simulink model "P3_model"  (R2023b)
settings: Solver=FixedStepAuto  StartTime=0.0  StopTime=240  FixedStep=0.01  RelTol=1e-3
values from neighbouring files (symbols this model uses):
  C0 = 0.0041    [init.m]
  C1 = 0.000066    (= 6.6e-05)    [init.m]
  C2 = 0.5*Rho*A*Cd    (= 0.51156)    [init.m]
  DriveData = DriveData_urban    [P3_runsim.m]
  Iw = 0.5*7*(r^2)    (= 0.4536)    [init.m]
  M = 1000    [init.m]
  mph2mps = 1600/3600    (= 0.444444444444)    [P3init.m]    (also in init.m)
  r = 0.36    [init.m]
  Time = (0:1:765)'    [init_HWY_DriveCycle.m]    (also in init_URB_DriveCycle.m = (0:1:1369)')
undefined symbols (not defined in the file or in its folder): carData
libraries: slpidlib x1
settings Model: Creator=anshu16  LastModifiedBy=jessi
settings SolverCC: AlgebraicLoopSolver=TrustRegion
settings OptimizationCC: ReuseModelBlockBuffer=off
settings DebuggingCC: UnconnectedInputMsg=warning  UnconnectedOutputMsg=warning  UnconnectedLineMsg=warning
settings ModelReferenceCC: EnableRefExpFcnMdlSchedulingChecks=on
settings SFSimCC: CustomCodeUndefinedFunction=UseInterfaceOnly

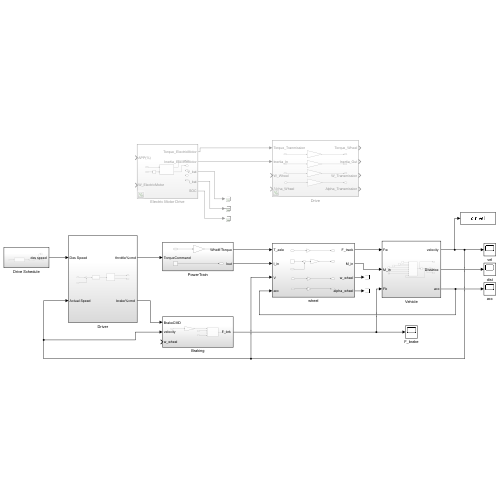
[thumbnail: Simulink's stored preview of the top-level diagram]
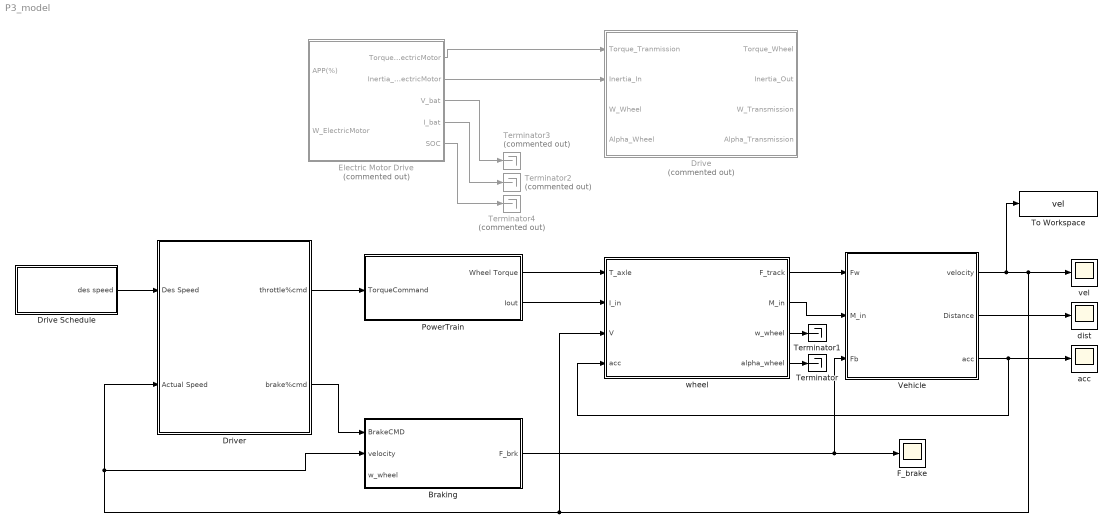
== system P3_model ==
  Braking : Subsystem
  Drive : Subsystem  Commented=on
  Drive Schedule : Subsystem
  "Driver " : Subsystem
  Electric Motor Drive : Subsystem  Commented=on
  F_brake : Scope
  PowerTrain : Subsystem
  Terminator : Terminator
  Terminator1 : Terminator
  Terminator2 : Terminator  Commented=on
  Terminator3 : Terminator  Commented=on
  Terminator4 : Terminator  Commented=on
  To Workspace : ToWorkspace  VariableName=vel  SaveFormat=Timeseries  SampleTime=-1
  Vehicle : Subsystem
  acc : Scope
  dist : Scope
  vel : Scope
  "wheel " : Subsystem
  wires:
  Drive Schedule/1("des speed ") -> "Driver "/1("Des Speed ")
  "Driver "/2("brake%cmd ") -> Braking/1("BrakeCMD ")
  Braking/1("F_brk ") -> Vehicle/3("Fb "), F_brake/1
  Vehicle/3(acc) -> acc/1, "wheel "/4(acc)
  PowerTrain/1(Wheel Torque) -> "wheel "/1(T_axle)
  PowerTrain/2(Iout) -> "wheel "/2(I_in)
  "wheel "/2(M_in) -> Vehicle/2("M_in ")
  "wheel "/1(F_track) -> Vehicle/1("Fw ")
  Vehicle/2("Distance ") -> dist/1
  Vehicle/1("velocity ") -> To Workspace/1, vel/1, "wheel "/3(V), "Driver "/2(Actual Speed), Braking/2("velocity ")
  "Driver "/1(throttle%cmd) -> PowerTrain/1(TorqueCommand)
  "wheel "/4(alpha_wheel) -> Terminator/1
  "wheel "/3(w_wheel) -> Terminator1/1
  Electric Motor Drive/3(V_bat) -> Terminator3/1
  Electric Motor Drive/4(I_bat) -> Terminator2/1
  Electric Motor Drive/5(SOC) -> Terminator4/1
  Electric Motor Drive/1(Torque_ElectricMotor) -> Drive/1(Torque_Tranmission)
  Electric Motor Drive/2(Inertia_ElectricMotor) -> Drive/2(Inertia_In)

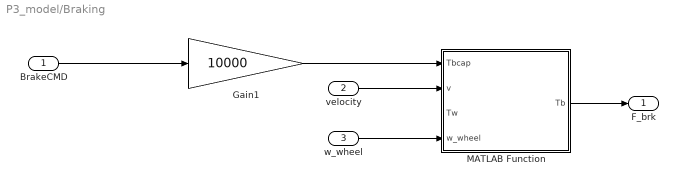
== system P3_model/Braking ==
  "BrakeCMD " : Inport
  "velocity " : Inport  Port=2
  w_wheel : Inport  Port=3
  Gain1 : Gain  Gain=10000
  MATLAB Function : MATLAB Function  TreatAsAtomicUnit=on
  "F_brk " : Outport  VectorParamsAs1DForOutWhenUnconnected=off
  wires:
  "BrakeCMD "/1 -> Gain1/1
  Gain1/1 -> MATLAB Function/1(Tbcap)
  MATLAB Function/1(Tb) -> "F_brk "/1
  "velocity "/1 -> MATLAB Function/2(v)
  w_wheel/1 -> MATLAB Function/4(w_wheel)

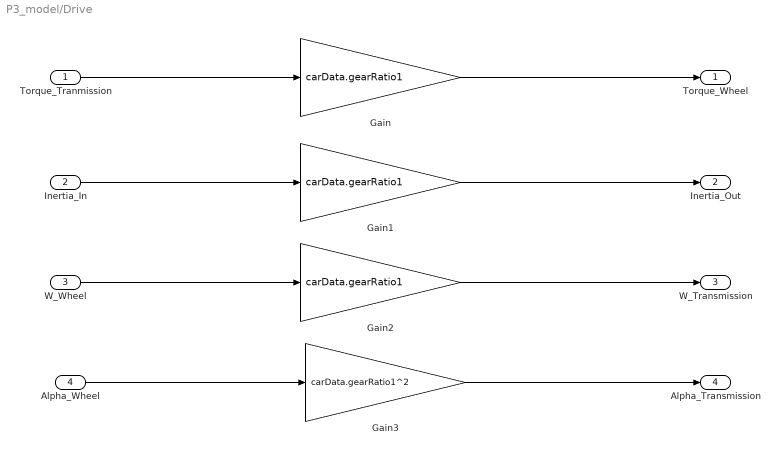
== system P3_model/Drive ==
  Torque_Tranmission : Inport
  Inertia_In : Inport  Port=2
  W_Wheel : Inport  Port=3
  Alpha_Wheel : Inport  Port=4
  Gain : Gain  Gain=carData.gearRatio1
  Gain1 : Gain  Gain=carData.gearRatio1
  Gain2 : Gain  Gain=carData.gearRatio1
  Gain3 : Gain  Gain=carData.gearRatio1^2
  Torque_Wheel : Outport
  Inertia_Out : Outport  Port=2
  W_Transmission : Outport  Port=3
  Alpha_Transmission : Outport  Port=4
  wires:
  Torque_Tranmission/1 -> Gain/1
  Inertia_In/1 -> Gain1/1
  W_Wheel/1 -> Gain2/1
  Alpha_Wheel/1 -> Gain3/1
  Gain/1 -> Torque_Wheel/1
  Gain1/1 -> Inertia_Out/1
  Gain2/1 -> W_Transmission/1
  Gain3/1 -> Alpha_Transmission/1

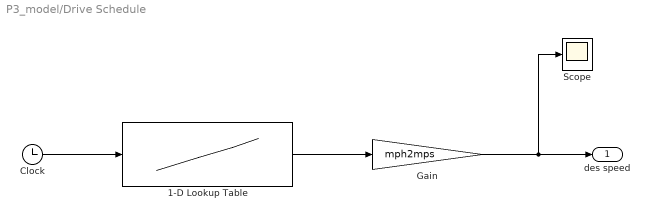
== system P3_model/Drive Schedule ==
  1-D Lookup Table : Lookup_n-D  NumberOfTableDimensions=1  BreakpointsForDimension1=Time  Table=DriveData  InternalRulePriority=Speed  RndMeth=Simplest
  Clock : Clock
  Gain : Gain  Gain=mph2mps
  Scope : Scope
  "des speed " : Outport  VectorParamsAs1DForOutWhenUnconnected=off
  wires:
  Clock/1 -> 1-D Lookup Table/1
  1-D Lookup Table/1 -> Gain/1
  Gain/1 -> "des speed "/1, Scope/1

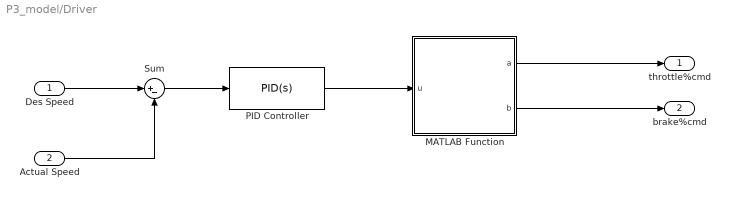
== system P3_model/Driver  ==
  "Des Speed " : Inport
  Actual Speed : Inport  Port=2
  MATLAB Function : MATLAB Function  TreatAsAtomicUnit=on
  PID Controller : slpidlib/PID Controller  Controller=PID  Form=Parallel  TimeDomain=Continuous-time  UseExternalTs=off  SampleTime=-1  IntegratorMethod=Forward Euler  FilterMethod=Forward Euler  ControllerParametersSource=internal  P=0.5  I=0  UseKiTs=off  D=0  N=100  UseFilter=on  TunerSelectOption=Transfer Function Based (PID Tuner App)  InitialConditionSource=internal  InitialConditionForIntegrator=0  InitialConditionForFilter=0  DifferentiatorICPrevScaledInput=0  ExternalReset=none  TrackingMode=off  Kt=1  LimitOutput=on  SatLimitsSource=internal  UpperSaturationLimit=1  LowerSaturationLimit=-1  LinearizeAsGain=off  AntiWindupMode=none  Kb=1  LimitIntegrator=off  UpperIntegratorSaturationLimit=inf  LowerIntegratorSaturationLimit=-inf  POutMin=[]  POutMax=[]  IOutMin=[]  IOutMax=[]  DOutMin=[]  DOutMax=[]  NOutMin=[]  NOutMax=[]  SumOutMin=[]  SumOutMax=[]  SaturationOutMin=[]  SaturationOutMax=[]  PParamMin=[]  PParamMax=[]  IParamMin=[]  IParamMax=[]  DParamMin=[]  DParamMax=[]  NParamMin=[]  NParamMax=[]  KbParamMin=[]  KbParamMax=[]  KtParamMin=[]  KtParamMax=[]  KbOutMin=[]  KbOutMax=[]  KtOutMin=[]  KtOutMax=[]  IntegratorOutMin=[]  IntegratorOutMax=[]  FilterOutMin=[]  FilterOutMax=[]  SumI1OutMin=[]  SumI1OutMax=[]  SumI2OutMin=[]  SumI2OutMax=[]  SumI3OutMin=[]  SumI3OutMax=[]  SumI4OutMin=[]  SumI4OutMax=[]  SumDOutMin=[]  SumDOutMax=[]  DifferentiatorOutMin=[]  DifferentiatorOutMax=[]  FilterDiffOutCoefMin=[]  FilterDiffOutCoefMax=[]  ReciprocalOutMin=[]  ReciprocalOutMax=[]  SumDenOutMin=[]  SumDenOutMax=[]  SumNumOutMin=[]  SumNumOutMax=[]  DivideOutMin=[]  DivideOutMax=[]  UdiffTsProdOutMin=[]  UdiffTsProdOutMax=[]  NTsProdOutMin=[]  NTsProdOutMax=[]  UintegralTsProdOutMin=[]  UintegralTsProdOutMax=[]  UngainTsProdOutMin=[]  UngainTsProdOutMax=[]  ClampingZeroOutDataTypeStr=Inherit: Inherit via back propagation  ClampingZeroOutMin=[]  ClampingZeroOutMax=[]  FilterDenConstantOutDataTypeStr=Inherit: Inherit via back propagation  FilterDenConstantOutMin=[]  FilterDenConstantOutMax=[]  PCopyOutDataTypeStr=Inherit: Inherit via back propagation  PCopyOutMin=[]  PCopyOutMax=[]  NCopyOutDataTypeStr=Inherit: Inherit via back propagation  NCopyOutMin=[]  NCopyOutMax=[]  IntegratorContinuousStateAttributes=''  IntegratorStateMustResolveToSignalObject=off  IntegratorRTWStateStorageClass=Auto  FilterContinuousStateAttributes=''  FilterStateMustResolveToSignalObject=off  FilterRTWStateStorageClass=Auto  ParallelPVariant=InternalParameters  IdealPVariant=Disabled  IVariant=InternalParameters  DVariant=InternalParameters  IntegratorVariant=Continuous  SatVariant=Enabled  AWVariant=Passthrough  PCopyVariant=Disabled  TRVariant=Disabled  FdbkBlocksVariant=Forward  IdealPFdbkVariant=Disabled  SatFdbkVariant=Disabled  DerivativeFilterVariant=ContFilter  NVariant=InternalParameters  NCopyVariant=Disabled  FilterICVariant=InternalICsFilter  IntegratorICVariant=InternalICs  ExternalResetVariant=Disabled  TRSumVariant=Passthrough  SumFdbkVariant=Disabled  SumVariant=Sum_PID  TsampFilterVariant=InternalTs  TsampNgainVariant=Passthrough  TsampIntegralVariant=Disabled_SignalSpec  ExternalSaturationOutDataTypeStr=Inherit: Same as second input
  Sum : Sum  Inputs=|+-
  throttle%cmd : Outport
  "brake%cmd " : Outport  Port=2
  wires:
  "Des Speed "/1 -> Sum/1
  Actual Speed/1 -> Sum/2
  MATLAB Function/2(b) -> "brake%cmd "/1
  MATLAB Function/1(a) -> throttle%cmd/1
  Sum/1 -> PID Controller/1
  PID Controller/1 -> MATLAB Function/1(u)

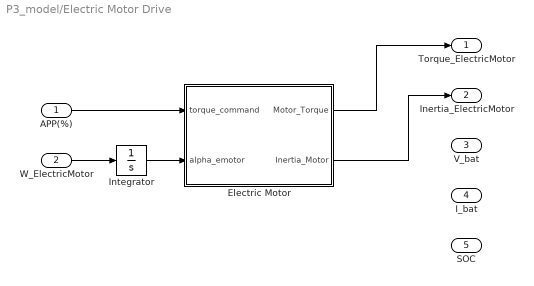
== system P3_model/Electric Motor Drive ==
  APP(%) : Inport
  W_ElectricMotor : Inport  Port=2
  Electric Motor : Subsystem
  Integrator : Integrator
  Torque_ElectricMotor : Outport
  Inertia_ElectricMotor : Outport  Port=2
  V_bat : Outport  Port=3
  I_bat : Outport  Port=4
  SOC : Outport  Port=5
  wires:
  Integrator/1 -> Electric Motor/2(alpha_emotor)
  W_ElectricMotor/1 -> Integrator/1
  APP(%)/1 -> Electric Motor/1(torque_command)
  Electric Motor/1(Motor_Torque) -> Torque_ElectricMotor/1
  Electric Motor/2(Inertia_Motor) -> Inertia_ElectricMotor/1

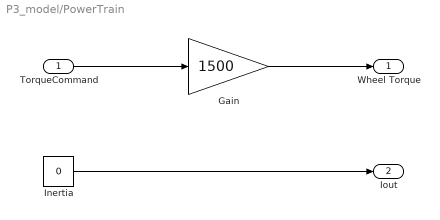
== system P3_model/PowerTrain ==
  TorqueCommand : Inport
  Gain : Gain  Gain=1500
  Inertia : Constant  Value=0
  Wheel Torque : Outport
  Iout : Outport  Port=2
  wires:
  TorqueCommand/1 -> Gain/1
  Gain/1 -> Wheel Torque/1
  Inertia/1 -> Iout/1

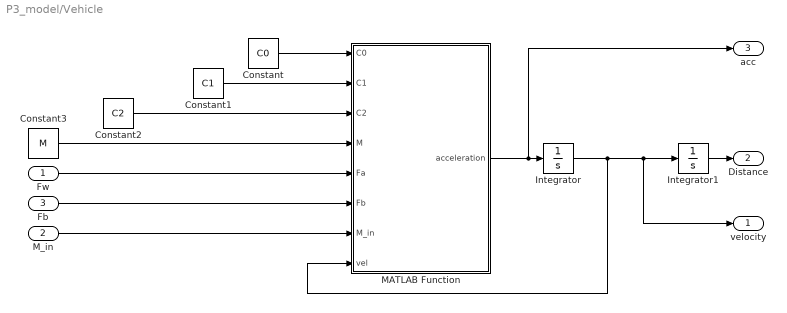
== system P3_model/Vehicle ==
  "Fw " : Inport
  "M_in " : Inport  Port=2
  "Fb " : Inport  Port=3
  Constant : Constant  Value=C0
  Constant1 : Constant  Value=C1
  Constant2 : Constant  Value=C2
  Constant3 : Constant  Value=M
  Integrator : Integrator  LimitOutput=on  LowerSaturationLimit=0
  Integrator1 : Integrator
  MATLAB Function : MATLAB Function  TreatAsAtomicUnit=on
  "velocity " : Outport  VectorParamsAs1DForOutWhenUnconnected=off
  "Distance " : Outport  Port=2  VectorParamsAs1DForOutWhenUnconnected=off
  acc : Outport  Port=3
  wires:
  Constant1/1 -> MATLAB Function/2(C1)
  Constant/1 -> MATLAB Function/1(C0)
  MATLAB Function/1(acceleration) -> acc/1, Integrator/1
  Constant2/1 -> MATLAB Function/3(C2)
  Constant3/1 -> MATLAB Function/4(M)
  "Fw "/1 -> MATLAB Function/5(Fa)
  "Fb "/1 -> MATLAB Function/6(Fb)
  Integrator/1 -> MATLAB Function/8(vel), "velocity "/1, Integrator1/1
  Integrator1/1 -> "Distance "/1
  "M_in "/1 -> MATLAB Function/7(M_in)

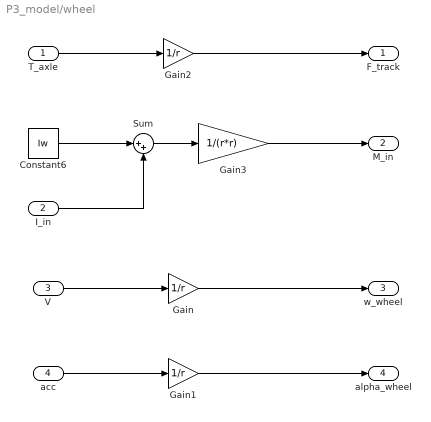
== system P3_model/wheel  ==
  T_axle : Inport
  I_in : Inport  Port=2
  V : Inport  Port=3
  acc : Inport  Port=4
  Constant6 : Constant  Value=Iw
  Gain : Gain  Gain=1/r
  Gain1 : Gain  Gain=1/r
  Gain2 : Gain  Gain=1/r
  Gain3 : Gain  Gain=1/(r*r)
  Sum : Sum  Inputs=|++
  F_track : Outport
  M_in : Outport  Port=2
  w_wheel : Outport  Port=3
  alpha_wheel : Outport  Port=4
  wires:
  Gain/1 -> w_wheel/1
  V/1 -> Gain/1
  acc/1 -> Gain1/1
  Gain1/1 -> alpha_wheel/1
  T_axle/1 -> Gain2/1
  Gain2/1 -> F_track/1
  Gain3/1 -> M_in/1
  Constant6/1 -> Sum/1
  I_in/1 -> Sum/2
  Sum/1 -> Gain3/1

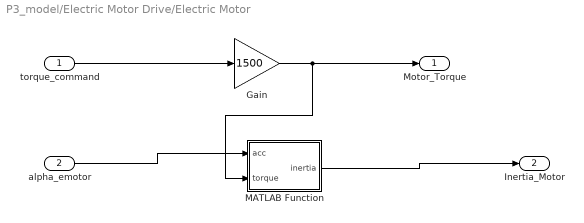
== system P3_model/Electric Motor Drive/Electric Motor ==
  torque_command : Inport
  alpha_emotor : Inport  Port=2
  Gain : Gain  Gain=1500
  MATLAB Function : MATLAB Function  TreatAsAtomicUnit=on
  Motor_Torque : Outport
  Inertia_Motor : Outport  Port=2
  wires:
  torque_command/1 -> Gain/1
  alpha_emotor/1 -> MATLAB Function/1(acc)
  Gain/1 -> MATLAB Function/2(torque), Motor_Torque/1
  MATLAB Function/1(inertia) -> Inertia_Motor/1

== matlab function P3_model/Driver /MATLAB Function ==
  data: u input; a output; b output
function [a,b] = fcn(u)

if u>0
    acc=u;
    brk=0;
elseif u<0
    acc=0;
    brk=-u;
else
    acc=0;
    brk=0;
end
a= acc;
b= brk;

== matlab function P3_model/Vehicle/MATLAB Function ==
  data: C0 input; acceleration output; C1 input; C2 input; M input; Fa input; Fb input; M_in input; vel input
function acceleration   = vehicle(C0,C1,C2,M,Fa,Fb,M_in, vel)

acceleration = (((Fa-Fb))-(C0+ C1*vel + C2*(vel)^2))/(M+M_in);


% Fa: Force from wheel.
% Fb: Force from brake.
% -(C0+ C1*vel + C2*(vel)^2)): Force from drag (opposite direction of motion)

== matlab function P3_model/Electric Motor Drive/Electric Motor/MATLAB Function ==
  data: acc input; inertia output; torque input
function inertia= fcn(acc, torque)

inertia = torque/acc;

== matlab function P3_model/Braking/MATLAB Function ==
  data: Tbcap input; Tb output; v input; Tw input; w_wheel input
function Tb = fcn(Tbcap, v, Tw,w_wheel)
Tb = Tbcap * v/(abs(v)+0.001);
end

% wrong, more logic needs to be added to this
% try to find where to incorporate Tw and w_wheel into function
